simulink model "MEDINP"  (R2022b)
settings: configuration reference "SharedConfig" (kept outside this file)
values from neighbouring files (symbols this model uses):
  DrvModReqDft_C : value not decoded    [MEDINP.sldd]
  DrvModReqDialEna_C = 1.0    [MEDINP.sldd]
  DrvModReqDialVal_C : value not decoded    [MEDINP.sldd]
  DT_MEDINP_C = 0.01    [MEDINP.sldd]
  McuReqTout_C = 0.07    [MEDINP.sldd]
  MotSpdReqCanDft_C = 0.0    [MEDINP.sldd]
  MotSpdReqCanDialEna_C = 1.0    [MEDINP.sldd]
  MotSpdReqCanDialVal_C = 0.0    [MEDINP.sldd]
  MotTqReqCanDft_C = 0.0    [MEDINP.sldd]
  MotTqReqCanDialEna_C = 1.0    [MEDINP.sldd]
  MotTqReqCanDialVal_C = 0.0    [MEDINP.sldd]
undefined symbols (not defined in the file or in its folder): DRIVEMODE, slcm
libraries: canmsglib x2, simulink x1, BlockLibrary x1
Description:
  | Converts raw inputs for the medium rate task into engineering units.
settings Model: DataDictionary=MEDINP.sldd  Creator=Kevin  LastModifiedBy=Max Kolesnikov
settings ConfigSetRef: SourceName=SharedConfig

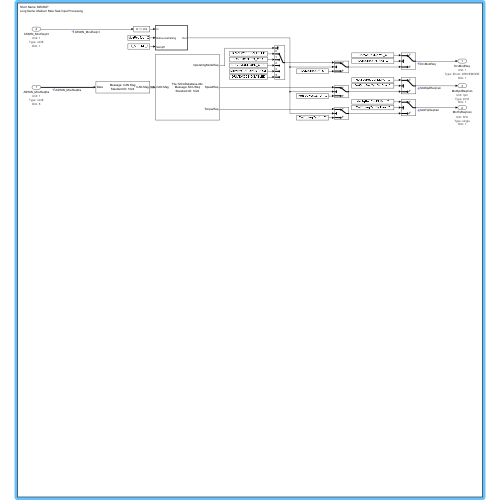
[thumbnail: Simulink's stored preview of the top-level diagram]
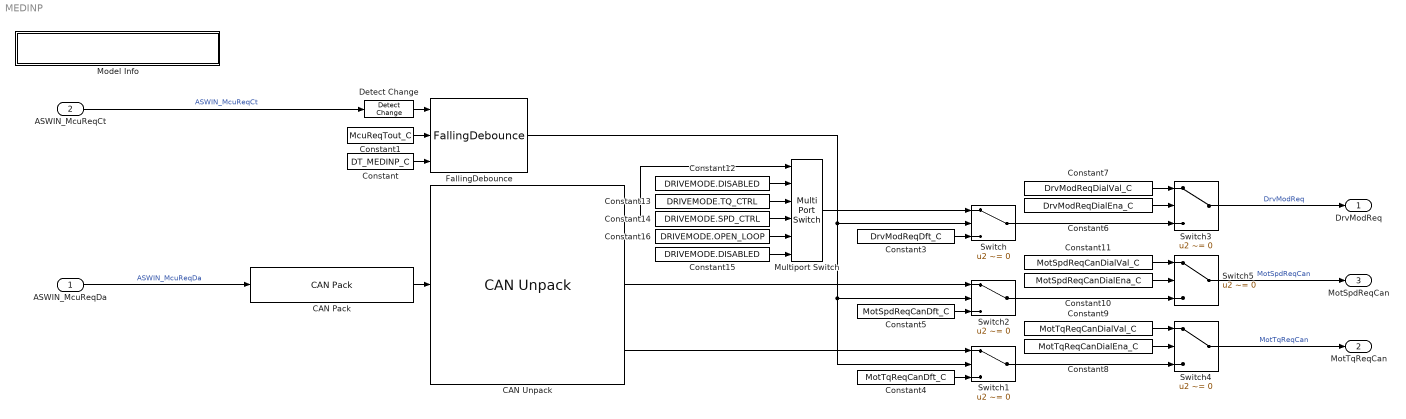
== system MEDINP ==
  ASWIN_McuReqDa : Inport  OutDataTypeStr=uint8  Unit=1  PortDimensions=8
      settings: AttributesFormatString=|
      | Unit: %<Unit>
      | Type: %<OutDataTypeStr>
      | Dim: %<PortDimensions>
  ASWIN_McuReqCt : Inport  Port=2  OutDataTypeStr=uint8  Unit=1  PortDimensions=1
      settings: AttributesFormatString=|
      | Unit: %<Unit>
      | Type: %<OutDataTypeStr>
      | Dim: %<PortDimensions>
  CAN Pack : canmsglib/CAN Pack  MsgList=(none)  MsgName=CAN Msg  MsgIDType=Standard (11-bit identifier)  MsgIdentifier=1024  MsgLength=8  Remote=off  ApplyMinMax=off  BusOutput=on  SignalInfo={}
      settings: LibrarySourceBlock=embeddedtargetslib/Host Communication/CAN Pack  DataFormat=raw data
  CAN Unpack : canmsglib/CAN Unpack  CANdbFile=C:\MKSTechRepos\P2319\p2319asw01\asw\lib\MCUDatabase.dbc  MsgList=MCUReq  MsgName=MCUReq  MsgIDType=Standard (11-bit identifier)  MsgIdentifier=1024  MsgLength=8  SignalInfo={'OperatingModeReq','0','2','LE','unsigned','Standard','0','1','0','-Inf','Inf';'SpeedReq','8','16','LE','unsigned','Standard','0','1','-32500','-32500','33035';'TorqueReq','24','16','LE','unsigned','Standard','0','0.1','-3250','-3250','3303.5'}  IDPort=off  TimestampPort=off  ErrorPort=off  RemotePort=off  LengthPort=off  StatusPort=off  ApplyMinMax=off
      settings: LibrarySourceBlock=embeddedtargetslib/Host Communication/CAN Unpack  DataFormat=CANdb specified signals
  Constant : Constant  Value=DT_MEDINP_C
  Constant1 : Constant  Value=McuReqTout_C
  Constant10 : Constant  Value=MotSpdReqCanDialEna_C
  Constant11 : Constant  Value=MotSpdReqCanDialVal_C
  Constant12 : Constant  Value=DRIVEMODE.DISABLED
  Constant13 : Constant  Value=DRIVEMODE.TQ_CTRL
  Constant14 : Constant  Value=DRIVEMODE.SPD_CTRL
  Constant15 : Constant  Value=DRIVEMODE.DISABLED
  Constant16 : Constant  Value=DRIVEMODE.OPEN_LOOP
  Constant3 : Constant  Value=DrvModReqDft_C
  Constant4 : Constant  Value=MotTqReqCanDft_C
  Constant5 : Constant  Value=MotSpdReqCanDft_C
  Constant6 : Constant  Value=DrvModReqDialEna_C
  Constant7 : Constant  Value=DrvModReqDialVal_C
  Constant8 : Constant  Value=MotTqReqCanDialEna_C
  Constant9 : Constant  Value=MotTqReqCanDialVal_C
  Detect Change : simulink/Logic and Bit Operations/Detect Change  vinit=0  OutDataTypeStr=boolean
  FallingDebounce : BlockLibrary/FallingDebounce  SystemSampleTime=-1  VariantActivationTime=update diagram  Latency=0  AutoFrameSizeCalculation=off
  Model Info : Subsystem  LoadFcn=slcm LoadBlock;  InitFcn=slcm('UpdateAllCMBlocksInThisModelInit')  mask(CMBlock){Frame=off, DisplayStringWithTags=|, MaskDisplayString=Short Name: MEDINP\nLong Name: Medium Rate Task Input Processing, HorizontalTextAlignment=Left, LeftAlignmentValue=0.02}
      mask DisplayStringWithTags=|
      | Short Name: %<ModelName>
      | Long Name: Medium Rate Task Input Processing
      mask prompts: Frame "Simulink:masks:Frame_MP"; DisplayStringWithTags "Simulink:masks:DisplayStringWithTags_MP"; MaskDisplayString "Simulink:masks:MaskDisplayString_MP"; HorizontalTextAlignment "Simulink:masks:HorizontalTextAlignment_MP"; LeftAlignmentValue "Simulink:masks:LeftAlignmentValue_MP"
      mask help: Simulink:masks:CMBlock_MD
      settings: CopyFcn=slcm CopyBlock;  DeleteFcn=slcm Cancel;  PostSaveFcn=slcm('UpdateAllCMBlocksInThisModel')  NameChangeFcn=slcm Rename;  OpenFcn=slcm
      mask Display: text(slResolve(LeftAlignmentValue, gcbh), 0.5, MaskDisplayString, 'HorizontalAlignment', HorizontalTextAlignment)
  Multiport Switch : MultiPortSwitch  DataPortOrder=Zero-based contiguous  Inputs=4  DataPortForDefault=Additional data port  DiagnosticForDefault=None  zeroidx=on  SaturateOnIntegerOverflow=off  InputSameDT=off
  Switch{,1..5} (6 alike) : Switch  Criteria=u2 ~= 0  SaturateOnIntegerOverflow=off  InputSameDT=off
  DrvModReq : Outport  OutDataTypeStr=Enum: DRIVEMODE  Unit=1  PortDimensions=1
      settings: AttributesFormatString=|
      | Unit: %<Unit>
      | Type: %<OutDataTypeStr>
      | Dim: %<PortDimensions>
  MotTqReqCan : Outport  Port=2  OutDataTypeStr=single  Unit=N*m  PortDimensions=1
      settings: AttributesFormatString=|
      | Unit: %<Unit>
      | Type: %<OutDataTypeStr>
      | Dim: %<PortDimensions>
  MotSpdReqCan : Outport  Port=3  OutDataTypeStr=int16  Unit=rpm  PortDimensions=1
      settings: AttributesFormatString=|
      | Unit: %<Unit>
      | Type: %<OutDataTypeStr>
      | Dim: %<PortDimensions>
  wires:
  Switch3/1 -> DrvModReq/1  "DrvModReq"
  CAN Pack/1 -> CAN Unpack/1
  ASWIN_McuReqDa/1 -> CAN Pack/1  "ASWIN_McuReqDa"
  ASWIN_McuReqCt/1 -> Detect Change/1  "ASWIN_McuReqCt"
  Detect Change/1 -> FallingDebounce/1
  FallingDebounce/1 -> Switch1/2, Switch2/2, Switch/2
  CAN Unpack/1 -> Multiport Switch/1
  Constant3/1 -> Switch/3
  Constant4/1 -> Switch1/3
  Constant5/1 -> Switch2/3
  Constant6/1 -> Switch3/2
  Constant7/1 -> Switch3/1
  Switch/1 -> Switch3/3
  Constant9/1 -> Switch4/1
  Constant8/1 -> Switch4/2
  Switch1/1 -> Switch4/3
  Constant10/1 -> Switch5/2
  Constant11/1 -> Switch5/1
  Switch2/1 -> Switch5/3
  Multiport Switch/1 -> Switch/1
  Constant12/1 -> Multiport Switch/2
  Constant13/1 -> Multiport Switch/3
  Constant14/1 -> Multiport Switch/4
  Constant15/1 -> Multiport Switch/6
  Switch4/1 -> MotTqReqCan/1  "MotTqReqCan"
  Switch5/1 -> MotSpdReqCan/1  "MotSpdReqCan"
  Constant16/1 -> Multiport Switch/5
  Constant1/1 -> FallingDebounce/2
  Constant/1 -> FallingDebounce/3
  CAN Unpack/2 -> Switch2/1
  CAN Unpack/3 -> Switch1/1

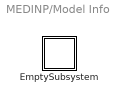
== system MEDINP/Model Info ==
  EmptySubsystem : Subsystem

== system MEDINP/Model Info/EmptySubsystem ==
